simulink model "SimulacionPasoR16"  (Simulink 8.9)
settings: Solver=ode45  StartTime=0.0  StopTime=10  RelTol=1e-3  EnableMultiTasking=on
values from neighbouring files (symbols this model uses):
  net = train(net,P,T)    [AplicacionIdentificacion.m]    (also in AplicacionIdentificacionTest.m)
undefined symbols (not defined in the file or in its folder): sim
settings Model: Creator=Helbert  LastModifiedBy=Helbert
settings OptimizationCC: InitFltsAndDblsToZero=on
settings DebuggingCC: SaveWithParameterizedLinksMsg=none  SignalResolutionControl=TryResolveAllWithWarning  SolverPrmCheckMsg=warning  MultiTaskDSMMsg=warning  MultiTaskCondExecSysMsg=none  FcnCallInpInsideContextMsg=error  StateNameClashWarn=none
settings GRTTargetCC: TargetFcnLib=ansi_tfl_tmw.mat  GeneratePreprocessorConditionals=Use local settings

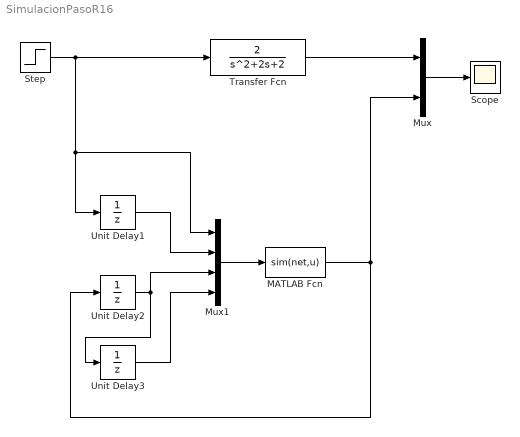
== system SimulacionPasoR16 ==
  MATLAB Fcn : MATLABFcn  MATLABFcn=sim(net,u)
  Mux : Mux  Inputs=2
  Mux1 : Mux
  Scope : Scope
  Step : Step  Time=0  SampleTime=0.1
  Transfer Fcn : TransferFcn  Numerator=[2]  Denominator=[1 2 2]
  Unit Delay1 : UnitDelay  SampleTime=0.1
  Unit Delay2 : UnitDelay  SampleTime=0.1
  Unit Delay3 : UnitDelay  SampleTime=0.1
  wires:
  Mux/1 -> Scope/1
  Step/1 -> Transfer Fcn/1, Unit Delay1/1, Mux1/1
  MATLAB Fcn/1 -> Mux/2, Unit Delay2/1
  Unit Delay2/1 -> Unit Delay3/1, Mux1/3
  Mux1/1 -> MATLAB Fcn/1
  Unit Delay1/1 -> Mux1/2
  Unit Delay3/1 -> Mux1/4
  Transfer Fcn/1 -> Mux/1
